simulink model "Plant2"  (R2022b)
settings: Solver=VariableStepAuto  StartTime=0.0  StopTime=1000  FixedStep=0.05  MaxStep=0.01  RelTol=1e-3
values from neighbouring files (symbols this model uses):
  phi = x(10)    [uav.m]    (also in uav1.m; uav2.m)
  psi = x(12)    [uav.m]    (also in uav1.m; uav2.m)
  r = length(idx)-1    [uav.m]    (also in uav1.m; uav2.m)
  theta = x(11)    [uav.m]    (also in uav1.m; uav2.m)
undefined symbols (not defined in the file or in its folder): airspeed, h_R, p, q, quat, timestamp, vd, ve, vn, x_R, y_R
libraries: simulink_extras x8, FC_Lib x2
settings Model: Creator=19114  LastModifiedBy=19114

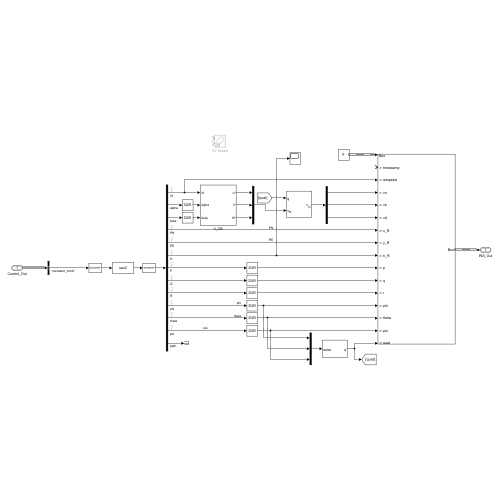
[thumbnail: Simulink's stored preview of the top-level diagram]
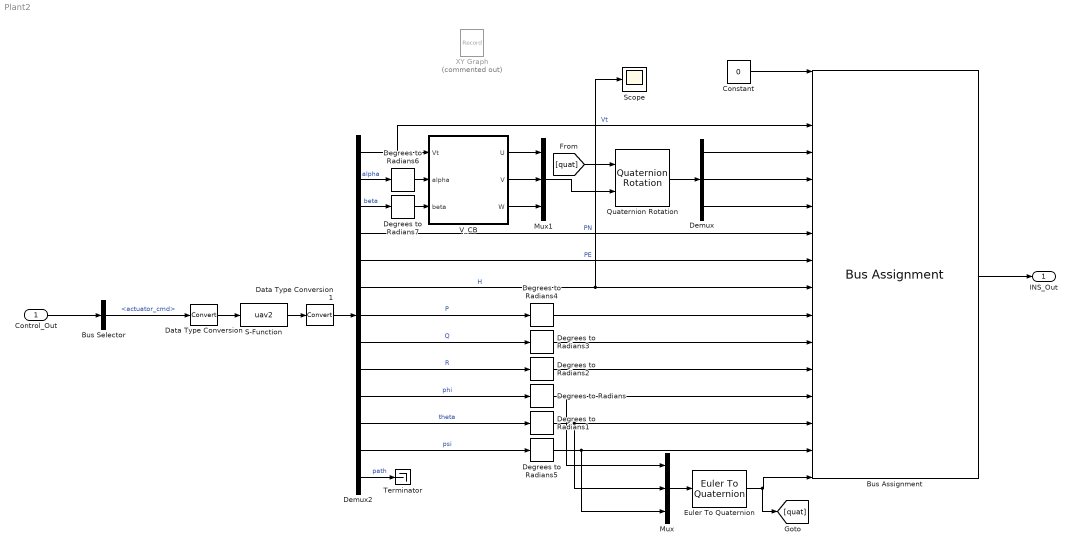
== system Plant2 ==
  Control_Out : Inport  OutDataTypeStr=Bus: Control_Out_Bus
  Bus Assignment : BusAssignment  AssignedSignals=timestamp,airspeed,vn,ve,vd,x_R,y_R,h_R,p,q,r,phi,theta,psi,quat
  Bus Selector : BusSelector  OutputSignals=actuator_cmd
  Constant : Constant  Value=0  OutDataTypeStr=Bus: INS_Out_Bus
  Data Type Conversion : DataTypeConversion  SaturateOnIntegerOverflow=off  RndMeth=Floor
  Data Type Conversion1 : DataTypeConversion  SaturateOnIntegerOverflow=off  RndMeth=Floor
  Degrees to Radians{,1..7} (8 alike) : simulink_extras/Transformations/Degrees to Radians
  Demux : Demux  Outputs=3
  Demux2 : Demux  Outputs=13
  Euler To Quaternion : FC_Lib/Quaternion/Euler To Quaternion
      settings: SourceProductName=Flight Control Toolbox
  Mux : Mux  Inputs=3
  Mux1 : Mux  Inputs=3
  Quaternion Rotation : FC_Lib/Quaternion/Quaternion Rotation
      settings: SourceProductName=Flight Control Toolbox
  S-Function : S-Function  FunctionName=uav2  SFunctionDeploymentMode=off  EnableBusSupport=off
  Scope : Scope
  Terminator : Terminator
  V_CB : Subsystem
  XY Graph : Record  Commented=on  FileSettingsInternal="{\"entries\":[{\"content\":{\"excelSettings\":{\"content\":{},\"type\":\"Streamout.ExcelSettings\"}},\"type\":\"Streamout.FileSettingStorage\",\"uuid\":\"\"}],\"packageUris\":[\"http:\\/\\/schema.mathworks.com\\/mf0\\/streamout_blocks\\/R2020a\"],\"version\":\"1.0\"}"  Layout=[1 1]  SignalsInternal="{\"entries\":[{\"content\":{\"signals\":[]},\"type\":\"RecordBlkView.InputSignals\",\"uuid\":\"\"}],\"packageUris\":[\"http:\\/\\/schema.mathworks.com\\/mf0\\/streamout_blocks\\/R2020a\"],\"version\":\"1.0\"}"  VisualizationBindings="{\"xyplotplugin\":{\"info\":[{\"series\":[],\"subplotID\":1}]}}"  CompatibilityTag=XY  st=-1
  INS_Out : Outport  OutDataTypeStr=Bus: INS_Out_Bus
  wires:
  Constant/1 -> Bus Assignment/1
  Bus Assignment/1 -> INS_Out/1
  Euler To Quaternion/1 -> [quat], Bus Assignment/16
  Degrees to Radians/1 -> Mux/1, Bus Assignment/13
  Mux/1 -> Euler To Quaternion/1
  Degrees to Radians1/1 -> Mux/2, Bus Assignment/14
  Demux/1 -> Bus Assignment/4
  Demux/3 -> Bus Assignment/6
  Demux/2 -> Bus Assignment/5
  Control_Out/1 -> Bus Selector/1
  Demux2/12 -> Degrees to Radians5/1  "psi"
  Demux2/13 -> Terminator/1  "path"
  Demux2/8 -> Degrees to Radians3/1  "Q"
  S-Function/1 -> Data Type Conversion1/1
  Demux2/10 -> Degrees to Radians/1  "phi"
  Demux2/9 -> Degrees to Radians2/1  "R"
  Bus Selector/1 -> Data Type Conversion/1  "<actuator_cmd>"
  Demux2/11 -> Degrees to Radians1/1  "theta"
  Demux2/7 -> Degrees to Radians4/1  "P"
  Demux2/4 -> Bus Assignment/7  "PN"
  Demux2/6 -> Scope/1, Bus Assignment/9  "H"
  Demux2/5 -> Bus Assignment/8  "PE"
  Data Type Conversion1/1 -> Demux2/1
  Data Type Conversion/1 -> S-Function/1
  Demux2/1 -> Bus Assignment/3, V_CB/1(Vt)  "Vt"
  Demux2/2 -> Degrees to Radians6/1  "alpha"
  Demux2/3 -> Degrees to Radians7/1  "beta"
  V_CB/1(U) -> Mux1/1
  V_CB/2(V) -> Mux1/2
  V_CB/3(W) -> Mux1/3
  Degrees to Radians2/1 -> Bus Assignment/12
  Degrees to Radians3/1 -> Bus Assignment/11
  Degrees to Radians4/1 -> Bus Assignment/10
  Degrees to Radians5/1 -> Mux/3, Bus Assignment/15
  Degrees to Radians6/1 -> V_CB/2(alpha)
  Degrees to Radians7/1 -> V_CB/3(beta)
  Quaternion Rotation/1 -> Demux/1
  [quat] -> Quaternion Rotation/1
  Mux1/1 -> Quaternion Rotation/2

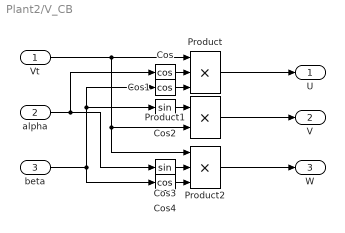
== system Plant2/V_CB ==
  Vt : Inport
  alpha : Inport  Port=2
  beta : Inport  Port=3
  Cos : Trigonometry  Operator=cos
  Cos1 : Trigonometry  Operator=cos
  Cos2 : Trigonometry
  Cos3 : Trigonometry
  Cos4 : Trigonometry  Operator=cos
  Product : Product  Inputs=3
  Product1 : Product
  Product2 : Product  Inputs=3
  U : Outport
  V : Outport  Port=2
  W : Outport  Port=3
  wires:
  Product1/1 -> V/1
  beta/1 -> Cos2/1, Cos1/1, Cos4/1
  Product/1 -> U/1
  Vt/1 -> Product1/2, Product2/1, Product/1
  Cos2/1 -> Product1/1
  Cos3/1 -> Product2/2
  alpha/1 -> Cos3/1, Cos/1
  Cos/1 -> Product/2
  Cos1/1 -> Product/3
  Cos4/1 -> Product2/3
  Product2/1 -> W/1
